simulink model "degree180_PWM"  (Simulink 7.9)
settings: Solver=ode45  StartTime=0.0  StopTime=inf  RelTol=1e-3
InitFcn:
  | Ts=5e-6;
undefined symbols (not defined in the file or in its folder): DiscIntNeverNeededParam
libraries: powerlib x15, powerlib_extras x3, simulink x2
settings Model: Creator=Abdul Rahman Kashif  LastModifiedBy=pleaseplease
settings DebuggingCC: FcnCallInpInsideContextMsg=Use local settings  StrictBusMsg=Warning
settings GRTTargetCC: CombineOutputUpdateFcns=off  GRTInterface=on

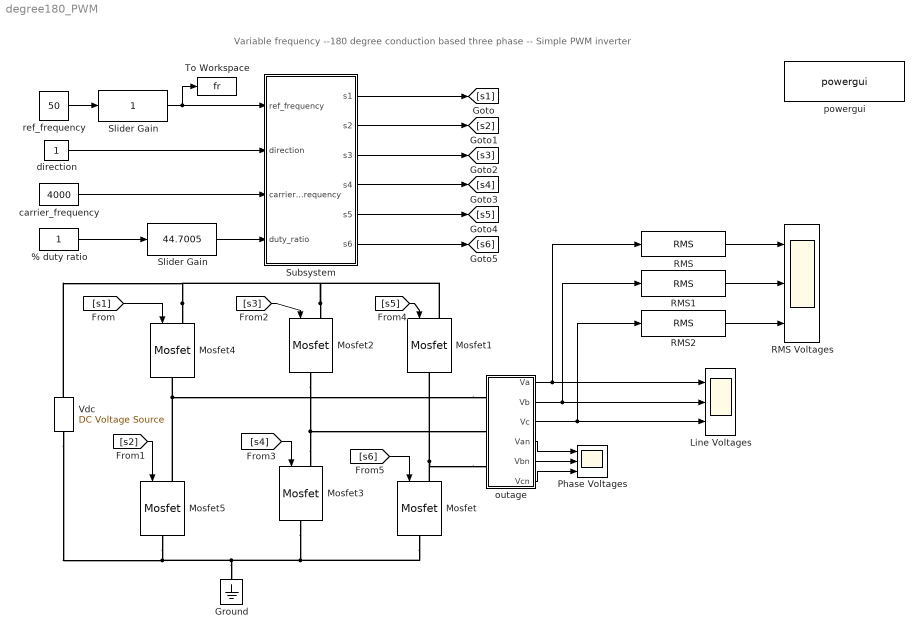
== system degree180_PWM ==
  note: Variable frequency --180 degree conduction based three phase -- Simple PWM inverter
  % duty ratio : Constant
  Ground : powerlib/Elements/Ground  LConnTagsString=a
  Line Voltages : Scope  NumInputPorts=3
      settings: TimeRange=0.1  YMin=-500~-500~-500  YMax=500~500~500  SaveName=Line_voltages  MaxDataPoints=50000  SampleInput=on  SampleTime=5e-6
  Mosfet{,1..5} (6 alike) : powerlib/Power Electronics/Mosfet  Ron=0.1  Lon=0  Rd=0.01  Vfd=0  IC=0  Rs=1e5  Cs=inf  Measurements=off
  Phase Voltages : Scope  NumInputPorts=3
      settings: TimeRange=0.1  YMin=-300~-300~-300  YMax=300~300~300  SaveName=Neutral_voltages  MaxDataPoints=50000  SampleInput=on  SampleTime=5e-6
  RMS : powerlib_extras/Measurements/RMS  f1=60
  RMS Voltages : Scope  NumInputPorts=3
      settings: TimeRange=0.1  YMin=200~210~210  YMax=232.5~227.5~227.5  SaveName=Neutral_voltages1  MaxDataPoints=50000  SampleInput=on  SampleTime=5e-6
  RMS1 : powerlib_extras/Measurements/RMS  f1=60
  RMS2 : powerlib_extras/Measurements/RMS  f1=60
  Slider Gain : simulink/Math Operations/Slider Gain  low=0  gain=1  high=4
  "Slider Gain  " : simulink/Math Operations/Slider Gain  low=0  gain=44.7005  high=100
  Subsystem : Subsystem
  To Workspace : ToWorkspace  VariableName=fr  SampleTime=-1  SaveFormat=Structure
  Vdc : powerlib/Electrical Sources/DC Voltage Source  Amplitude=400  Measurements=None
  carrier_frequency : Constant  Value=4000
  direction : Constant
  outage : Subsystem
  powergui : powerlib/powergui  Priority=1  SimulationMode=Discrete  SolverType=Tustin  SampleTime=Ts  frequency=60  SPID=off  DisableSnubberDevices=off  DisableRonSwitches=off  DisableVfSwitches=off  SwTol=0  Interpol=off  DisplayEquations=off  FunctionMessages=off  frequencyindice=0  Pbase=100e6  ErrMax=1e-4  Iterations=50  UnitsV=kV  UnitsW=MW  echomessages=off  HookPort=off  EnableUseOfTLC=off  x0status=blocks  RestoreLinks=warning  ResistiveCurrentMeasurement=off  Frange=[0:2:500]  Ylog=off  Xlog=on  ShowGrid=off  save=off  variable=ZData  structure=Line_voltages  ZoomFFT=off  StartTime=1.4  cycles=5  DisplayStyle=2  fundamental=fr  FreqAxis=off  MaxFrequency=1000  frequencyindicesteady=1  RmsSteady=1  display=off  Ts=0  methode=off
  ref_frequency : Constant  Value=50
  wires:
  ref_frequency/1 -> Slider Gain/1
  direction/1 -> Subsystem/2(direction)
  [s1] -> Mosfet4/1
  [s2] -> Mosfet5/1
  [s3] -> Mosfet2/1
  [s4] -> Mosfet3/1
  [s5] -> Mosfet1/1
  [s6] -> Mosfet/1
  outage/4(Van) -> Phase Voltages/1
  outage/5(Vbn) -> Phase Voltages/2
  outage/6(Vcn) -> Phase Voltages/3
  Subsystem/1(s1) -> [s1]
  Subsystem/2(s2) -> [s2]
  Subsystem/3(s3) -> [s3]
  Subsystem/4(s4) -> [s4]
  Subsystem/5(s5) -> [s5]
  Subsystem/6(s6) -> [s6]
  Slider Gain/1 -> Subsystem/1(ref_frequency), To Workspace/1
  outage/1(Va) -> Line Voltages/1, RMS/1
  outage/2(Vb) -> Line Voltages/2, RMS1/1
  outage/3(Vc) -> Line Voltages/3, RMS2/1
  carrier_frequency/1 -> Subsystem/3(carrier_frequency)
  % duty ratio/1 -> "Slider Gain  "/1
  "Slider Gain  "/1 -> Subsystem/4(duty_ratio)
  RMS/1 -> RMS Voltages/1
  RMS1/1 -> RMS Voltages/2
  RMS2/1 -> RMS Voltages/3
  connections:
  Vdc/RConn1 -- Mosfet4/LConn1 -- Mosfet2/LConn1 -- Mosfet1/LConn1
  outage/LConn1 -- Mosfet4/RConn1 -- Mosfet5/LConn1
  outage/LConn3 -- Mosfet/LConn1 -- Mosfet1/RConn1
  Ground/LConn1 -- Mosfet/RConn1 -- Mosfet3/RConn1 -- Vdc/LConn1 -- Mosfet5/RConn1
  Mosfet3/LConn1 -- outage/LConn2 -- Mosfet2/RConn1

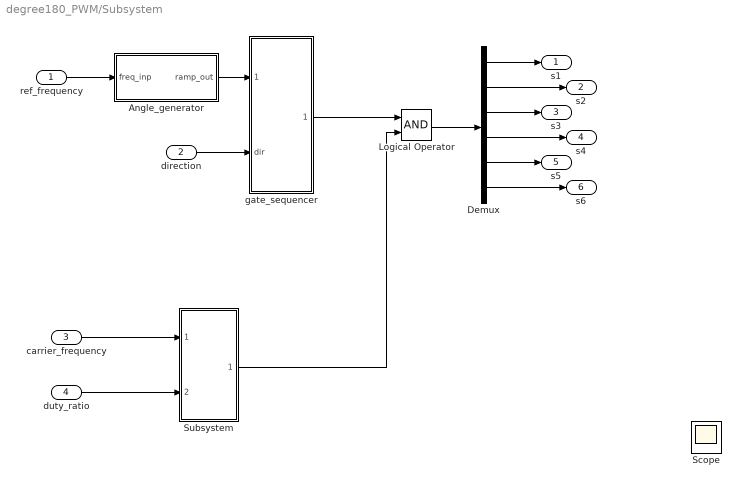
== system degree180_PWM/Subsystem ==
  ref_frequency : Inport
  direction : Inport  Port=2
  carrier_frequency : Inport  Port=3
  duty_ratio : Inport  Port=4
  Angle_generator : Subsystem
  Demux : Demux  Outputs=6
  Logical Operator : Logic  AllPortsSameDT=off  OutDataTypeStr=boolean
  Scope : Scope  NumInputPorts=3
      settings: YMin=-5~-5~-5  YMax=5~5~5  MaxDataPoints=5000000
  Subsystem : Subsystem
  gate_sequencer : Subsystem
  s1 : Outport
  s2 : Outport  Port=2
  s3 : Outport  Port=3
  s4 : Outport  Port=4
  s5 : Outport  Port=5
  s6 : Outport  Port=6
  wires:
  Angle_generator/1(ramp_out) -> gate_sequencer/1(ramp_inp)
  Demux/1 -> s1/1
  ref_frequency/1 -> Angle_generator/1(freq_inp)
  Demux/2 -> s2/1
  Demux/3 -> s3/1
  Demux/4 -> s4/1
  Demux/5 -> s5/1
  direction/1 -> gate_sequencer/2(dir)
  Demux/6 -> s6/1
  carrier_frequency/1 -> Subsystem/1(carrier_frequency)
  duty_ratio/1 -> Subsystem/2(%duty_ratio)
  gate_sequencer/1(gate_logic) -> Logical Operator/1
  Subsystem/1(PWM_signal) -> Logical Operator/2
  Logical Operator/1 -> Demux/1

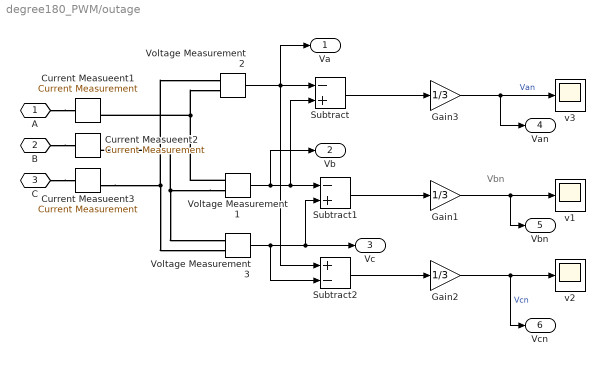
== system degree180_PWM/outage ==
  note: Vbn
  Current Measueent1 : powerlib/Measurements/Current Measurement  PhasorSimulation=off  OutputType=Complex  PSBequivalent=0
  Current Measueent2 : powerlib/Measurements/Current Measurement  PhasorSimulation=off  OutputType=Complex  PSBequivalent=0
  Current Measueent3 : powerlib/Measurements/Current Measurement  PhasorSimulation=off  OutputType=Complex  PSBequivalent=0
  Gain1 : Gain  Gain=1/3
  Gain2 : Gain  Gain=1/3
  Gain3 : Gain  Gain=1/3
  Subtract : Sum  Inputs=-+
  Subtract1 : Sum  Inputs=-+
  Subtract2 : Sum  Inputs=+-
  Voltage Measurement1 : powerlib/Measurements/Voltage Measurement  PhasorSimulation=off  OutputType=Complex  PSBequivalent=0
  Voltage Measurement2 : powerlib/Measurements/Voltage Measurement  PhasorSimulation=off  OutputType=Complex  PSBequivalent=0
  Voltage Measurement3 : powerlib/Measurements/Voltage Measurement  PhasorSimulation=off  OutputType=Complex  PSBequivalent=0
  v1 : Scope
      settings: SaveName=ScopeData25  MaxDataPoints=5000000
  v2 : Scope
      settings: SaveName=ScopeData26  MaxDataPoints=5000000
  v3 : Scope
      settings: YMin=-300  YMax=300  SaveName=ScopeData27  MaxDataPoints=5000000
  A : PMIOPort  Port=1  Side=Left
  B : PMIOPort  Port=2  Side=Left
  C : PMIOPort  Port=3  Side=Left
  Va : Outport
  Vb : Outport  Port=2
  Vc : Outport  Port=3
  Van : Outport  Port=4
  Vbn : Outport  Port=5
  Vcn : Outport  Port=6
  wires:
  Gain2/1 -> v2/1, Vcn/1  "Vcn"
  Subtract2/1 -> Gain2/1
  Gain1/1 -> v1/1, Vbn/1
  Subtract1/1 -> Gain1/1
  Voltage Measurement3/1 -> Subtract2/2, Subtract1/2, Vc/1
  Gain3/1 -> v3/1, Van/1  "Van"
  Subtract/1 -> Gain3/1
  Voltage Measurement1/1 -> Subtract/2, Subtract1/1, Vb/1
  Voltage Measurement2/1 -> Subtract/1, Subtract2/1, Va/1
  connections:
  Voltage Measurement1/LConn1 -- Current Measueent1/RConn1 -- Voltage Measurement2/LConn2
  Voltage Measurement1/LConn2 -- Current Measueent2/RConn1 -- Voltage Measurement3/LConn1
  Current Measueent3/RConn1 -- Voltage Measurement2/LConn1 -- Voltage Measurement3/LConn2
  A/RConn1 -- Current Measueent1/LConn1
  B/RConn1 -- Current Measueent2/LConn1
  C/RConn1 -- Current Measueent3/LConn1

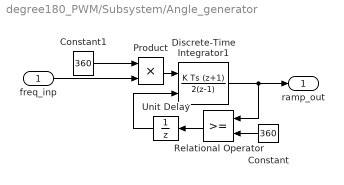
== system degree180_PWM/Subsystem/Angle_generator ==
  freq_inp : Inport
  Constant : Constant  Value=360
  Constant1 : Constant  Value=360
  Discrete-Time Integrator1 : DiscreteIntegrator  IntegratorMethod=Integration: Trapezoidal  ExternalReset=rising  SampleTime=Ts  ICPrevOutput=DiscIntNeverNeededParam  ICPrevScaledInput=DiscIntNeverNeededParam
  Product : Product  SaturateOnIntegerOverflow=on  InputSameDT=on  OutDataTypeStr=Inherit: Same as first input
  Relational Operator : RelationalOperator  InputSameDT=on
  Unit Delay : UnitDelay  SampleTime=Ts
  ramp_out : Outport
  wires:
  Discrete-Time Integrator1/1 -> Relational Operator/1, ramp_out/1
  Constant/1 -> Relational Operator/2
  Relational Operator/1 -> Unit Delay/1
  Unit Delay/1 -> Discrete-Time Integrator1/2
  Constant1/1 -> Product/1
  Product/1 -> Discrete-Time Integrator1/1
  freq_inp/1 -> Product/2

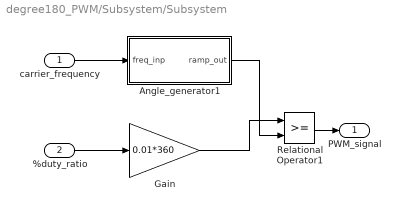
== system degree180_PWM/Subsystem/Subsystem ==
  carrier_frequency : Inport
  %duty_ratio : Inport  Port=2
  Angle_generator1 : Subsystem
  Gain : Gain  Gain=0.01*360
  Relational Operator1 : RelationalOperator  InputSameDT=on
  PWM_signal : Outport
  wires:
  Gain/1 -> Relational Operator1/1
  Angle_generator1/1(ramp_out) -> Relational Operator1/2
  carrier_frequency/1 -> Angle_generator1/1(freq_inp)
  Relational Operator1/1 -> PWM_signal/1
  %duty_ratio/1 -> Gain/1

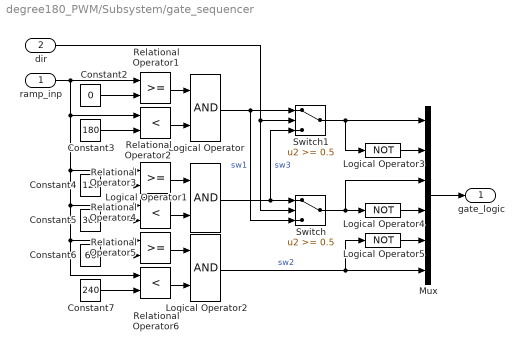
== system degree180_PWM/Subsystem/gate_sequencer ==
  ramp_inp : Inport
  dir : Inport  Port=2
  Constant2 : Constant  Value=0
  Constant3 : Constant  Value=180
  Constant4 : Constant  Value=120
  Constant5 : Constant  Value=300
  Constant6 : Constant  Value=60
  Constant7 : Constant  Value=240
  Logical Operator : Logic
  Logical Operator1 : Logic
  Logical Operator2 : Logic
  Logical Operator3 : Logic  Operator=NOT
  Logical Operator4 : Logic  Operator=NOT
  Logical Operator5 : Logic  Operator=NOT
  Mux : Mux  Inputs=6
  Relational Operator1 : RelationalOperator  InputSameDT=on
  Relational Operator2 : RelationalOperator  Operator=<  InputSameDT=on
  Relational Operator3 : RelationalOperator  InputSameDT=on
  Relational Operator4 : RelationalOperator  Operator=<  InputSameDT=on
  Relational Operator5 : RelationalOperator  InputSameDT=on
  Relational Operator6 : RelationalOperator  Operator=<  InputSameDT=on
  Switch : Switch  Threshold=0.5  SaturateOnIntegerOverflow=on  InputSameDT=on
  Switch1 : Switch  Threshold=0.5  SaturateOnIntegerOverflow=on  InputSameDT=on
  gate_logic : Outport
  wires:
  Constant4/1 -> Relational Operator3/2
  Constant5/1 -> Relational Operator4/2
  Relational Operator3/1 -> Logical Operator1/1
  Relational Operator4/1 -> Logical Operator1/2
  Constant6/1 -> Relational Operator5/2
  Constant7/1 -> Relational Operator6/2
  Relational Operator5/1 -> Logical Operator2/1
  Relational Operator6/1 -> Logical Operator2/2
  Logical Operator3/1 -> Mux/2
  Logical Operator4/1 -> Mux/4
  Logical Operator5/1 -> Mux/5
  Logical Operator2/1 -> Logical Operator5/1, Mux/6  "sw2"
  Logical Operator/1 -> Switch1/1, Switch/3  "sw1"
  Mux/1 -> gate_logic/1
  Switch1/1 -> Mux/1, Logical Operator3/1
  Switch/1 -> Logical Operator4/1, Mux/3
  dir/1 -> Switch1/2, Switch/2
  Logical Operator1/1 -> Switch/1, Switch1/3  "sw3"
  Constant2/1 -> Relational Operator1/2
  Constant3/1 -> Relational Operator2/2
  Relational Operator1/1 -> Logical Operator/1
  Relational Operator2/1 -> Logical Operator/2
  ramp_inp/1 -> Relational Operator1/1, Relational Operator2/1, Relational Operator3/1, Relational Operator4/1, Relational Operator5/1, Relational Operator6/1

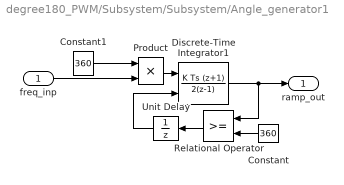
== system degree180_PWM/Subsystem/Subsystem/Angle_generator1 ==
  freq_inp : Inport
  Constant : Constant  Value=360
  Constant1 : Constant  Value=360
  Discrete-Time Integrator1 : DiscreteIntegrator  IntegratorMethod=Integration: Trapezoidal  ExternalReset=rising  SampleTime=Ts  ICPrevOutput=DiscIntNeverNeededParam  ICPrevScaledInput=DiscIntNeverNeededParam
  Product : Product  SaturateOnIntegerOverflow=on  InputSameDT=on  OutDataTypeStr=Inherit: Same as first input
  Relational Operator : RelationalOperator  InputSameDT=on
  Unit Delay : UnitDelay  SampleTime=Ts
  ramp_out : Outport
  wires:
  Discrete-Time Integrator1/1 -> Relational Operator/1, ramp_out/1
  Constant/1 -> Relational Operator/2
  Relational Operator/1 -> Unit Delay/1
  Unit Delay/1 -> Discrete-Time Integrator1/2
  Constant1/1 -> Product/1
  Product/1 -> Discrete-Time Integrator1/1
  freq_inp/1 -> Product/2
